simulink model "Lab_6"  (R2024b)
settings: Solver=ode3  StartTime=0.0  StopTime=1500  FixedStep=0.5  RelTol=1e-3  EnableMultiTasking=on
libraries: arduinolib x2
settings Model: ExtModeTrigDuration=2  Creator=ANUSHKA  LastModifiedBy=Acer
settings DataIOCC: SaveOutput=off  DSMLogging=off  SaveTime=off  ReturnWorkspaceOutputs=off
settings OptimizationCC: EnhancedBackFolding=on  PassReuseOutputArgsAs=Individual arguments  ZeroExternalMemoryAtStartup=off  ZeroInternalMemoryAtStartup=off  MaxStackSize=64  OptimizeBlockOrder=speed  DifferentSizesBufferReuse=on  OptimizationCustomize=off  EfficientTunableParamExpr=on
settings DebuggingCC: ParameterTunabilityLossMsg=error
settings HardwareCC: ProdBitPerInt=16  ProdBitPerPointer=16  ProdBitPerSizeT=16  ProdBitPerPtrDiffT=16  ProdLargestAtomicFloat=None  ProdWordSize=8  ProdHWDeviceType=Atmel->AVR
settings SFSimCC: MATLABDynamicMemAlloc=off
settings RTWCC: Description=Embedded Coder  SystemTargetFile=ert.tlc  HardwareBoard=Arduino Uno  TemplateMakefile=ert_default_tmf  Toolchain=Arduino AVR  BuildConfiguration=Faster Runs
settings CodeAppCC: ForceParamTrailComments=on  IgnoreCustomStorageClasses=off  OperatorAnnotations=on  SimulinkDataObjDesc=on  SFDataObjDesc=on  InsertBlockDesc=on
settings ERTTargetCC: SupportContinuousTime=on  SupportVariableSizeSignals=on  ExtModeTransport=3  ExtModeStaticAlloc=on  ExtModeAutomaticAllocSize=off  ExtModeStaticAllocSize=250  ExtModeMexFile=ext_xcp  ExtModeIntrfLevel=Level2 - Open  InlinedParameterPlacement=Hierarchical

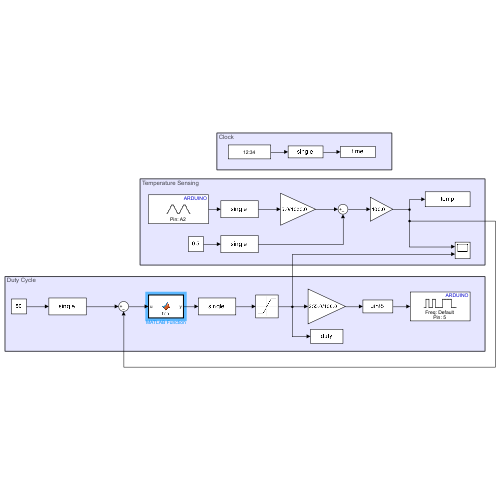
[thumbnail: Simulink's stored preview of the top-level diagram]
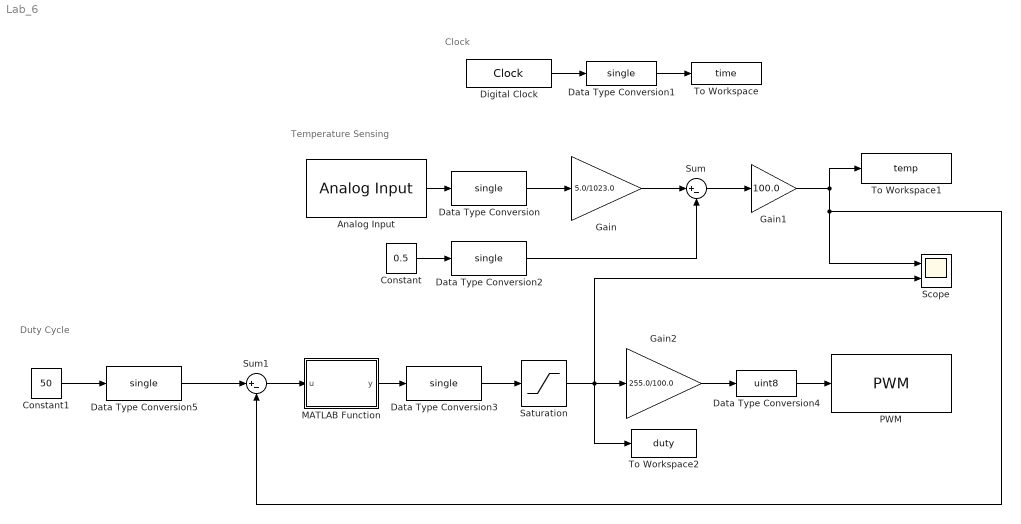
== system Lab_6 ==
  note: Duty Cycle
  note: Temperature Sensing
  note: Clock
  Analog Input : arduinolib/Analog Input  pinNumber=2  ReadResultsOnly=off  ConversionTriggerSource=Software  ExternalTriggerType=uint32( 0 )  OutputDataType=uint16  EnableConversionCompleteNotify=off  EnableOuputStatus=off  SampleTime=0.5  blockPlatform=arduino
  Constant : Constant  Value=0.5
  Constant1 : Constant  Value=50
  Data Type Conversion{,1..3,5} (5 alike) : DataTypeConversion  OutDataTypeStr=single  SaturateOnIntegerOverflow=off  RndMeth=Floor
  Data Type Conversion4 : DataTypeConversion  OutDataTypeStr=uint8  SaturateOnIntegerOverflow=off  RndMeth=Floor
  Digital Clock : DigitalClock  SampleTime=0.5
  Gain : Gain  Gain=5.0/1023.0
  Gain1 : Gain  Gain=100.0
  Gain2 : Gain  Gain=255.0/100.0
  MATLAB Function : MATLAB Function  TreatAsAtomicUnit=on
  PWM : arduinolib/PWM  pinNumber=5  frequencyType=Default  desiredFrequency=490.2  achievableFrequency=490.2
  Saturation : Saturate  UpperLimit=100  LowerLimit=0
  Scope : Scope  NumInputPorts=2
  Sum : Sum  Inputs=|+-
  Sum1 : Sum  Inputs=|+-
  To Workspace : ToWorkspace  VariableName=time  SampleTime=0.5
  To Workspace1 : ToWorkspace  VariableName=temp  SampleTime=0.5
  To Workspace2 : ToWorkspace  VariableName=duty  SampleTime=0.5
  wires:
  Analog Input/1 -> Data Type Conversion/1
  Data Type Conversion/1 -> Gain/1
  Digital Clock/1 -> Data Type Conversion1/1
  Data Type Conversion1/1 -> To Workspace/1
  Gain/1 -> Sum/1
  Constant/1 -> Data Type Conversion2/1
  Data Type Conversion2/1 -> Sum/2
  Sum/1 -> Gain1/1
  Gain1/1 -> To Workspace1/1, Sum1/2, Scope/1
  MATLAB Function/1(y) -> Data Type Conversion3/1
  Data Type Conversion3/1 -> Saturation/1
  Saturation/1 -> To Workspace2/1, Scope/2, Gain2/1
  Gain2/1 -> Data Type Conversion4/1
  Data Type Conversion4/1 -> PWM/1
  Constant1/1 -> Data Type Conversion5/1
  Data Type Conversion5/1 -> Sum1/1
  Sum1/1 -> MATLAB Function/1(u)

== matlab function Lab_6/MATLAB Function ==
  data: u input; y output
function y = fcn(u)

if (u>=20.0)
    y = 40.0 + 50.0;
elseif (u>=10.0) & (u<20.0)
    y = 20.0 + 50.0;
elseif (u>=0.0) & (u<10.0)
    y = 10.0 + 50.0;
else
    y = 0.0+50.0;

end
